simulink model "MotorPos"  (R2020b)
settings: Solver=ode45  StartTime=0.0  StopTime=0.2  RelTol=1e-3
undefined symbols (not defined in the file or in its folder): Kd, Ki, Kp
settings Model: DataDictionary=DataDictionary.sldd  SimulationMode=accelerator  PacingRate=1000000  Creator=abhin  LastModifiedBy=abhin
settings SolverCC: InitialStep=0.0001  AlgebraicLoopSolver=LineSearch

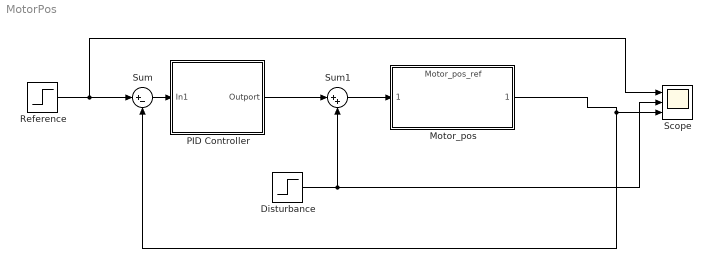
== system MotorPos ==
  Disturbance : Step  Time=0.03  SampleTime=0
  Motor_pos : ModelReference  ModelNameDialog=Motor_pos_ref  SimulationMode=Normal  ModelReferenceVersion=1.6
  PID Controller : Subsystem
  Reference : Step  Time=0  SampleTime=0
  Scope : Scope  NumInputPorts=3
  Sum : Sum  Inputs=|+-
  Sum1 : Sum  Inputs=|++
  wires:
  Motor_pos/1 -> Sum/2, Scope/3
  Reference/1 -> Scope/1, Sum/1
  Sum1/1 -> Motor_pos/1
  Disturbance/1 -> Sum1/2, Scope/2
  Sum/1 -> PID Controller/1(In1)
  PID Controller/1(Outport) -> Sum1/1

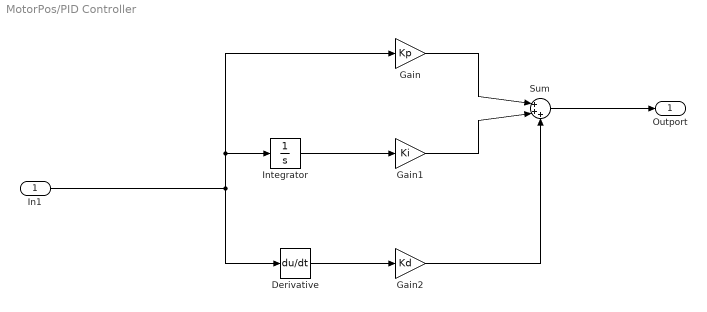
== system MotorPos/PID Controller ==
  In1 : Inport
  Derivative : Derivative
  Gain : Gain  Gain=Kp
  Gain1 : Gain  Gain=Ki
  Gain2 : Gain  Gain=Kd
  Integrator : Integrator
  Sum : Sum  Inputs=|+++
  Outport : Outport
  wires:
  Gain2/1 -> Sum/3
  Gain/1 -> Sum/1
  In1/1 -> Derivative/1, Integrator/1, Gain/1
  Gain1/1 -> Sum/2
  Sum/1 -> Outport/1
  Integrator/1 -> Gain1/1
  Derivative/1 -> Gain2/1
